simulink model "model"  (R2023b)
settings: Solver=VariableStepAuto  StartTime=0.0  StopTime=6  RelTol=1e-3
undefined symbols (not defined in the file): k, T_m, U_pr
settings Model: Creator=m  LastModifiedBy=m

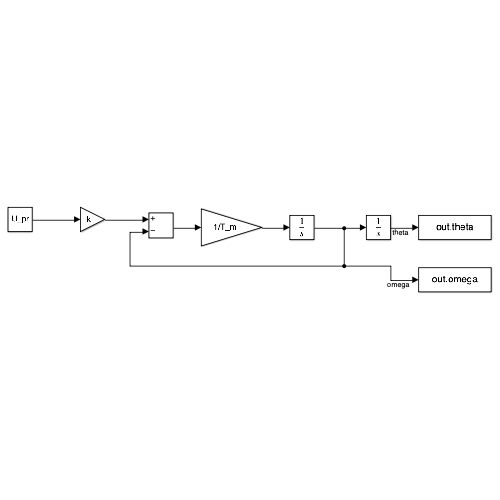
[thumbnail: Simulink's stored preview of the top-level diagram]
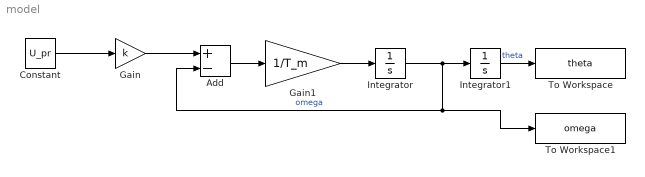
== system model ==
  Add : Sum  Inputs=+-
  Constant : Constant  Value=U_pr
  Gain : Gain  Gain=k
  Gain1 : Gain  Gain=1/T_m
  Integrator : Integrator
  Integrator1 : Integrator
  To Workspace : ToWorkspace  VariableName=theta  SaveFormat=Timeseries  SampleTime=-1
  To Workspace1 : ToWorkspace  VariableName=omega  SaveFormat=Timeseries  SampleTime=-1
  wires:
  Constant/1 -> Gain/1
  Gain/1 -> Add/1
  Add/1 -> Gain1/1
  Gain1/1 -> Integrator/1
  Integrator/1 -> To Workspace1/1, Add/2, Integrator1/1  "omega"
  Integrator1/1 -> To Workspace/1  "theta"
